simulink model "example"  (Simulink 6.6)
settings: Solver=FixedStepDiscrete  StartTime=0.0  StopTime=inf  FixedStep=0.01  RelTol=1e-3
settings Model: Creator=Jon Mills  LastModifiedBy=Jon Mills  CovMetricSettings=dcw
settings DataIOCC: LimitDataPoints=off  SaveOutput=off  SignalLogging=off  SaveTime=off
settings OptimizationCC: BooleanDataType=off
settings DebuggingCC: SignalResolutionControl=TryResolveAllWithWarning  SolverPrmCheckMsg=none  MultiTaskDSMMsg=warning  MultiTaskCondExecSysMsg=none  StrictBusMsg=None
settings HardwareCC: TargetUnknown=on
settings RTWCC: IncludeERTFirstTime=on

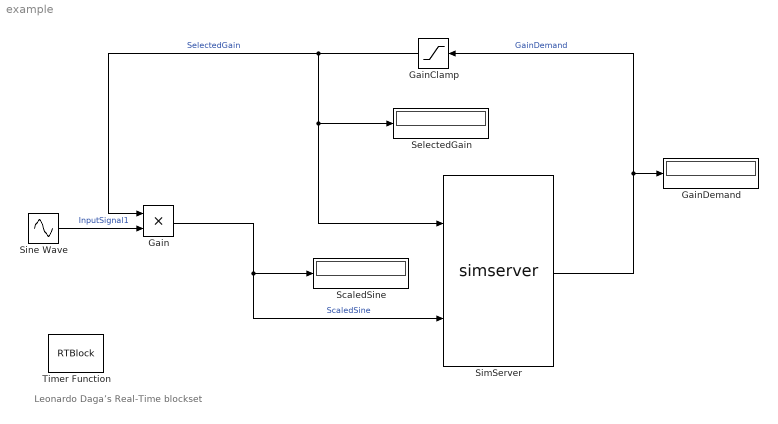
== system example ==
  note: Leonardo Daga’s Real-Time blockset
  Gain : Product  RndMeth=Zero
  GainClamp : Saturate  Orientation=left  UpperLimit=10  LowerLimit=1
  GainDemand : Display
  ScaledSine : Display
  SelectedGain : Display
  SimServer : S-Function  Description=Modbus client  FunctionName=simserver  Parameters=80,'io_config.cfg',gcb
  Sine Wave : Sin  SampleTime=0.01
  Timer Function : S-Function  FunctionName=RTBlock  Parameters=step,rtpriority,ThPriority  mask(RTBlock){step=50, rtpriority=HIGH, ThPriority=TIME CRITICAL}
      mask prompts: step "Timestep (ms)"; rtpriority "Priority"; ThPriority "Thread Priority"
      mask help:
      | Real Time Block: Set the characteristics of a real-time simulation. The settings of the simulation are selectable using the block panel. The parameters are:
      |
      | - Timeout: in milliseconds, defines the temporization with which Simulink requires to the Operating System the availability of resources for the execution of the simulation step. The value should be fixed equal to the simulation step of Simulink (the timestep);
      |
      | - Priority Class: defines the class of task priority required, that can be one of the following values:
      | -- IDLE PRIORITY: Low priority, typical of an idle process (priority less than normal)
      | -- NORMAL PRIORITY: Typical priority of a typical windows application;
      | -- HIGH PRIORITY: Typical priority of a relevant application, that needs more resources of a normal application;
      | -- REAL-TIME PRIORITY: Exclusive priority of a unique process that needs all the resources of the operating system.
      |
      | - Thread Priority: defines the class of task priority required, that can be one of the following values:
      | -- IDLE : The thread should run when the main process is inactive.
      | -- LOWEST : The thread runs with a minimal respect of the temporization;
      | -- NORMAL : The thread runs with the same priority of the main process;
      | -- HIGH : The thread runs with the major priority respect to the main process;
      | -- REAL-TIME : The process runs when the simulation thread is in idle state.
      mask StyleString: edit,popup(IDLE|NORMAL|HIGH|REAL-TIME),popup(IDLE|LOWEST|NORMAL|HIGHEST|TIME CRITICAL)
  wires:
  SimServer/1 -> GainDemand/1, GainClamp/1  "GainDemand"
  Sine Wave/1 -> Gain/2  "InputSignal1"
  GainClamp/1 -> Gain/1, SimServer/1, SelectedGain/1  "SelectedGain"
  Gain/1 -> SimServer/2, ScaledSine/1  "ScaledSine"
